simulink model "linearesModell"  (R2017b)
settings: Solver=VariableStepAuto  StartTime=0.0  StopTime=10.0  RelTol=1e-3
values from neighbouring files (symbols this model uses):
  A1 = [0 1 0 0 ... (first row only)    [StartSim.m]
  A2 = [0 1 ; 0 -1/T2]    [StartSim.m]
  B1 = [0 b2 0 b4]'    [StartSim.m]
  B2 = [0  2*pi*r2*K2/(ue2*T2)]'    [StartSim.m]
  C1 = eye(4)    [StartSim.m]
  C2 = eye(2)    [StartSim.m]
  D1 = [0 0 0 0]'    [StartSim.m]
  D2 = [0 0]'    [StartSim.m]
  L_0 = 0.2    [StartSim.m]
  phi_0 = 0    [StartSim.m]
  x_0 = 0    [StartSim.m]
undefined symbols (not defined in the file or in its folder): t01, t02, t1, t2, u1, u2
settings Model: Creator=Patrick  LastModifiedBy=Patrick

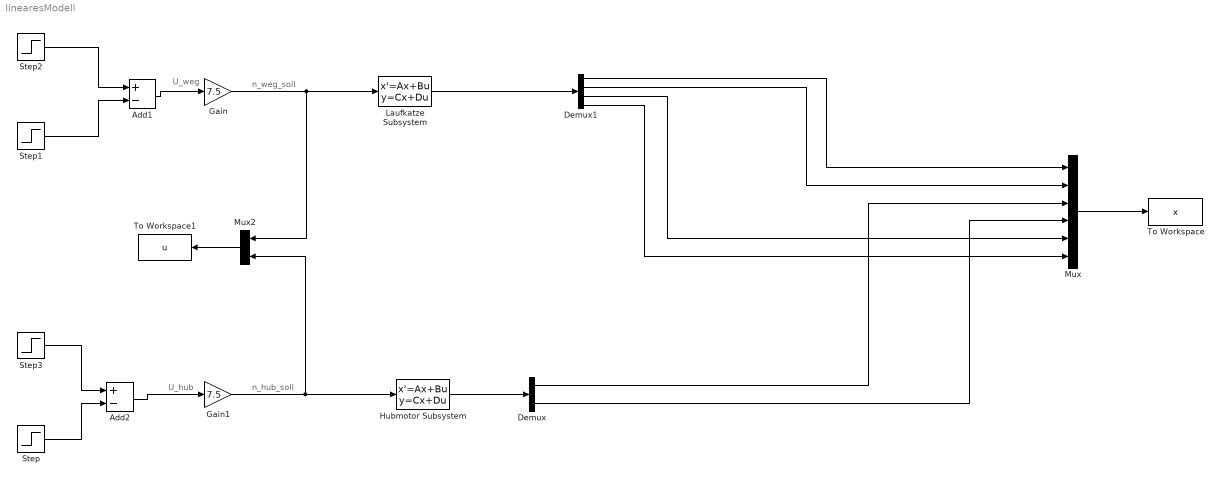
== system linearesModell ==
  note: n_weg_soll
  note: U_weg
  note: n_hub_soll
  note: U_hub
  Add1 : Sum  Inputs=+-
  Add2 : Sum  Inputs=+-
  Demux : Demux  Outputs=2
  Demux1 : Demux
  Gain : Gain  Gain=7.5
  Gain1 : Gain  Gain=7.5
  Hubmotor Subsystem : StateSpace  A=A2  B=B2  C=C2  D=D2  InitialCondition=[L_0 ; 0]
  Laufkatze Subsystem : StateSpace  A=A1  B=B1  C=C1  D=D1  InitialCondition=[x_0 ; 0 ; phi_0 ; 0]
  Mux : Mux  Inputs=6
  Mux2 : Mux  Inputs=2
  Step : Step  Time=t2  After=u2  SampleTime=0
  Step1 : Step  Time=t1  After=u1  SampleTime=0
  Step2 : Step  Time=t01  After=u1  SampleTime=0
  Step3 : Step  Time=t02  After=u2  SampleTime=0
  To Workspace : ToWorkspace  VariableName=x  SampleTime=-1
  To Workspace1 : ToWorkspace  VariableName=u  SampleTime=-1
  wires:
  Add1/1 -> Gain/1
  Gain/1 -> Laufkatze Subsystem/1, Mux2/1
  Step1/1 -> Add1/2
  Step2/1 -> Add1/1
  Gain1/1 -> Hubmotor Subsystem/1, Mux2/2
  Add2/1 -> Gain1/1
  Mux2/1 -> To Workspace1/1
  Step/1 -> Add2/2
  Step3/1 -> Add2/1
  Hubmotor Subsystem/1 -> Demux/1
  Mux/1 -> To Workspace/1
  Laufkatze Subsystem/1 -> Demux1/1
  Demux1/1 -> Mux/1
  Demux1/2 -> Mux/2
  Demux1/3 -> Mux/5
  Demux1/4 -> Mux/6
  Demux/1 -> Mux/3
  Demux/2 -> Mux/4
